simulink model "psbcurrmeasure"  (Simulink 6.0)
settings: Solver=ode23s  SolverMode=SingleTasking  StartTime=0.0  StopTime=0.1  RelTol=1e-3  AbsTol=1e-6
libraries: powerlib2 x15
settings Model: Creator=patrice  LastModifiedBy=batserve  ExtModeTrigMode=oneshot  ExtModeArmWhenConnect=off  ExtModeAutoUpdateStatusClock=off
settings DataIOCC: LimitDataPoints=off  SignalLoggingName=sigsOut
settings OptimizationCC: BooleanDataType=off
settings DebuggingCC: SolverPrmCheckMsg=none
settings HardwareCC: TargetUnknown=on
settings RTWCC: TemplateMakefile=grt_unix.tmf

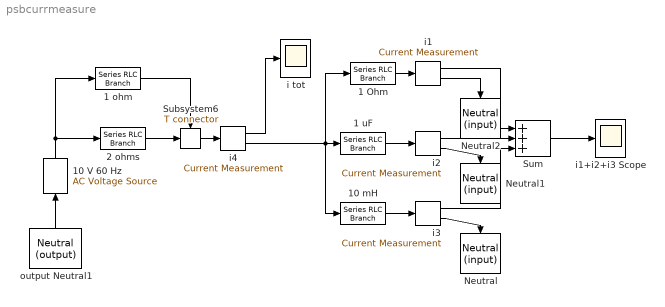
== system psbcurrmeasure ==
  1 Ohm : powerlib2/Elements/Series RLC Branch  Tag=PoWeRsYsTeMbLoCk  a=1  b=0  c=inf  mesure=None  PSBOutputType=1
  1 ohm : powerlib2/Elements/Series RLC Branch  Tag=PoWeRsYsTeMbLoCk  a=1  b=0  c=inf  mesure=None  PSBOutputType=1
  1 uF : powerlib2/Elements/Series RLC Branch  Tag=PoWeRsYsTeMbLoCk  a=0  b=0  c=1e-6  mesure=None  PSBOutputType=1
  10 V 60 Hz : powerlib2/Electrical Sources/AC Voltage Source  Tag=PoWeRsYsTeMbLoCk  Orientation=up  A=10  P=0  F=60  stime=0  mesure=None  PSBOutputType=1
  10 mH : powerlib2/Elements/Series RLC Branch  Tag=PoWeRsYsTeMbLoCk  a=0  b=10  c=inf  mesure=None  PSBOutputType=1
  2 ohms : powerlib2/Elements/Series RLC Branch  Tag=PoWeRsYsTeMbLoCk  a=2  b=0  c=inf  mesure=None  PSBOutputType=1
  Neutral : powerlib2/Connectors/Neutral (input)  Tag=PoWeRsYsTeMbLoCk  Orientation=down  no=50
  Neutral1 : powerlib2/Connectors/Neutral (input)  Tag=PoWeRsYsTeMbLoCk  Orientation=down  no=50
  Neutral2 : powerlib2/Connectors/Neutral (input)  Tag=PoWeRsYsTeMbLoCk  Orientation=down  no=50
  Subsystem6 : powerlib2/Connectors/T connector  Tag=PoWeRsYsTeMbLoCk  PSBOutputType=1
  Sum : Sum  Inputs=+++  SaturateOnIntegerOverflow=on  InputSameDT=on
  i tot : Scope
      settings: TickLabels=on  TimeRange=0.1  YMin=-12  YMax=12  DataFormat=Array
  i{1..4} (4 alike) : powerlib2/Measurements/Current Measurement  Tag=PoWeRsYsTeMmEaSuReMeNt  PhasorSimulation=off  OutputType=Magnitude  PSBOutputType=01  PSBequivalent=0
  i1+i2+i3 Scope : Scope
      settings: TickLabels=on  TimeRange=0.1  YMin=-12  YMax=12  DataFormat=Array
  output Neutral1 : powerlib2/Connectors/Neutral (output)  Tag=PoWeRsYsTeMbLoCk  Orientation=up  no=50  PSBOutputType=1
  wires:
  10 V 60 Hz/1 -> 1 ohm/1, 2 ohms/1
  output Neutral1/1 -> 10 V 60 Hz/1
  1 ohm/1 -> Subsystem6/Enable
  2 ohms/1 -> Subsystem6/1
  Subsystem6/1 -> i4/1
  i4/1 -> i tot/1
  i4/2 -> 1 uF/1, 1 Ohm/1, 10 mH/1
  i3/2 -> Neutral/1
  i3/1 -> Sum/3
  i2/2 -> Neutral1/1
  i2/1 -> Sum/2
  i1/2 -> Neutral2/1
  i1/1 -> Sum/1
  1 uF/1 -> i2/1
  1 Ohm/1 -> i1/1
  10 mH/1 -> i3/1
  Sum/1 -> i1+i2+i3 Scope/1
